simulink model "quadsim2009"  (Simulink 7.7)
settings: Solver=ode45  StartTime=0.0  StopTime=50  RelTol=1e-3
values from neighbouring files (symbols this model uses):
  b = 9.7575e-6    (= 9.7575e-06)    [ForcesTest.m]    (also in QuadDynamics.m = 9.937e-09; QuadDynamicsC.m = 1.7246e-06; Quadparameters.m = 3.13e-05; quadparam.m = 3.13e-05)
  d = 7.5*10^(-7)    (= 7.5e-07)    [Quadparameters.m]    (also in quadparam.m)
  g = 9.81    [ForcesTest.m]    (also in QuadDynamics.m; QuadDynamicsC.m; Quadparameters.m; quadparam.m)
  Ix = 7.5*10^(-3)    (= 0.0075)    [Quadparameters.m]    (also in quadparam.m)
  Iy = 7.5*10^(-3)    (= 0.0075)    [Quadparameters.m]    (also in quadparam.m)
  Iz = 1.3*10^(-2)    (= 0.013)    [Quadparameters.m]    (also in quadparam.m)
  Jr = 6.5*10^(-5)    (= 6.5e-05)    [Quadparameters.m]    (also in quadparam.m = 0.100065)
  kdp = 0.4    [Quadparameters.m]    (also in quadparam.m)
  kdps = 0.4    [Quadparameters.m]    (also in quadparam.m)
  kdt = 0.4    [Quadparameters.m]    (also in quadparam.m)
  kdz = 20    [Quadparameters.m]    (also in quadparam.m = 80)
  kpp = 0.8    [Quadparameters.m]    (also in quadparam.m)
  kpps = 1    [Quadparameters.m]    (also in quadparam.m)
  kpt = 1.2    [Quadparameters.m]    (also in quadparam.m)
  kpz = 100    [Quadparameters.m]    (also in quadparam.m)
  l = 0.3    [ForcesTest.m]    (also in QuadDynamics.m = 0.254; QuadDynamicsC.m = 0.254; Quadparameters.m = 0.23; quadparam.m = 0.5)
  m = 1.282    [ForcesTest.m]    (also in QuadDynamics.m = 1.284; QuadDynamicsC.m = 1.284; Quadparameters.m = 0.65; quadparam.m = 0.65)
libraries: simulink x2
settings Model: Creator=abdelrazzak.merheb  LastModifiedBy=Alexey
settings DebuggingCC: StrictBusMsg=Warning

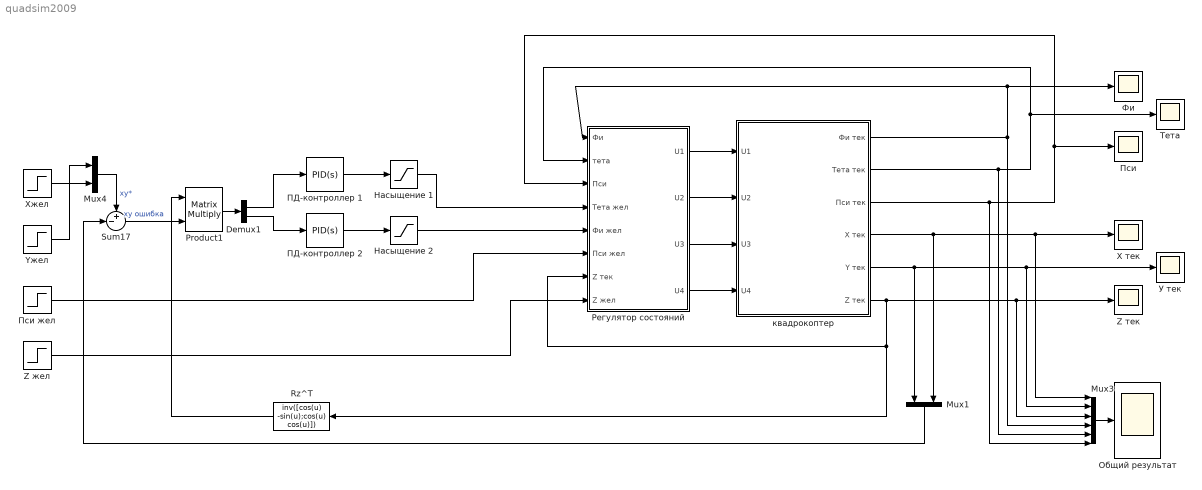
== system quadsim2009 ==
  Demux1 : Demux  Outputs=2
  Mux1 : Mux  Inputs=2
  Mux3 : Mux  Inputs=6
  Mux4 : Mux  Inputs=2
  Product1 : Product  Multiplication=Matrix(*)  RndMeth=Zero
  Rz^T : MATLABFcn  MATLABFcn=inv([cos(u) -sin(u);cos(u) cos(u)])  OutputDimensions=[2 2]  Output1D=off
  Sum17 : Sum  Inputs=+-|
  X тек : Scope
      settings: TimeRange=50  YMin=-0.02  YMax=0.08  SaveName=ScopeData6
  Xжел : Step  Time=10  After=2  SampleTime=0
  Yжел : Step  After=4  SampleTime=0
  Z жел : Step  After=20  SampleTime=0
  Z тек : Scope
      settings: TimeRange=50  YMin=0  YMax=1.4  SaveName=ScopeData4
  Насыщение 1 : Saturate  LinearizeAsGain=off
  Насыщение 2 : Saturate
  Общий результат : Scope
      settings: SaveName=ScopeData3
  ПД-контроллер 1 : simulink/Continuous/PID Controller  SystemSampleTime=-1  Controller=PID  TimeDomain=Continuous-time  SampleTime=1  IntegratorMethod=Forward Euler  FilterMethod=Forward Euler  Form=Parallel  P=1  I=0.1  D=2  N=100  InitialConditionSource=internal  InitialConditionForIntegrator=0  InitialConditionForFilter=0  ExternalReset=none  LimitOutput=off  UpperSaturationLimit=inf  LowerSaturationLimit=-inf  LinearizeAsGain=off  AntiWindupMode=none  Kb=1  TrackingMode=off  Kt=1  PParamMin=[]  PParamMax=[]  IParamMin=[]  IParamMax=[]  DParamMin=[]  DParamMax=[]  NParamMin=[]  NParamMax=[]  KbParamMin=[]  KbParamMax=[]  KtParamMin=[]  KtParamMax=[]  POutMin=[]  POutMax=[]  IOutMin=[]  IOutMax=[]  DOutMin=[]  DOutMax=[]  NOutMin=[]  NOutMax=[]  KbOutMin=[]  KbOutMax=[]  KtOutMin=[]  KtOutMax=[]  IntegratorOutMin=[]  IntegratorOutMax=[]  FilterOutMin=[]  FilterOutMax=[]  SumOutMin=[]  SumOutMax=[]  SumI1OutMin=[]  SumI1OutMax=[]  SumI2OutMin=[]  SumI2OutMax=[]  SumI3OutMin=[]  SumI3OutMax=[]  SumDOutMin=[]  SumDOutMax=[]  SaturationOutMin=[]  SaturationOutMax=[]  IntegratorContinuousStateAttributes=''  IntegratorStateMustResolveToSignalObject=off  IntegratorRTWStateStorageClass=Auto  FilterContinuousStateAttributes=''  FilterStateMustResolveToSignalObject=off  FilterRTWStateStorageClass=Auto
  ПД-контроллер 2 : simulink/Continuous/PID Controller  SystemSampleTime=-1  Controller=PID  TimeDomain=Continuous-time  SampleTime=1  IntegratorMethod=Forward Euler  FilterMethod=Forward Euler  Form=Parallel  P=1  I=0.1  D=2  N=100  InitialConditionSource=internal  InitialConditionForIntegrator=0  InitialConditionForFilter=0  ExternalReset=none  LimitOutput=off  UpperSaturationLimit=inf  LowerSaturationLimit=-inf  LinearizeAsGain=off  AntiWindupMode=none  Kb=1  TrackingMode=off  Kt=1  PParamMin=[]  PParamMax=[]  IParamMin=[]  IParamMax=[]  DParamMin=[]  DParamMax=[]  NParamMin=[]  NParamMax=[]  KbParamMin=[]  KbParamMax=[]  KtParamMin=[]  KtParamMax=[]  POutMin=[]  POutMax=[]  IOutMin=[]  IOutMax=[]  DOutMin=[]  DOutMax=[]  NOutMin=[]  NOutMax=[]  KbOutMin=[]  KbOutMax=[]  KtOutMin=[]  KtOutMax=[]  IntegratorOutMin=[]  IntegratorOutMax=[]  FilterOutMin=[]  FilterOutMax=[]  SumOutMin=[]  SumOutMax=[]  SumI1OutMin=[]  SumI1OutMax=[]  SumI2OutMin=[]  SumI2OutMax=[]  SumI3OutMin=[]  SumI3OutMax=[]  SumDOutMin=[]  SumDOutMax=[]  SaturationOutMin=[]  SaturationOutMax=[]  IntegratorContinuousStateAttributes=''  IntegratorStateMustResolveToSignalObject=off  IntegratorRTWStateStorageClass=Auto  FilterContinuousStateAttributes=''  FilterStateMustResolveToSignalObject=off  FilterRTWStateStorageClass=Auto
  Пси : Scope
      settings: YMin=1.08342  YMax=1.08355
  Пси жел : Step  After=0  SampleTime=0
  Регулятор состояний : Subsystem
  Тета : Scope
      settings: TimeRange=30  YMin=-0.5  YMax=2  SaveName=ScopeData2
  У тек : Scope
      settings: TimeRange=30  YMin=-0.5  YMax=2  SaveName=ScopeData7
  Фи : Scope
      settings: TimeRange=50  YMax=25
  квадрокоптер : Subsystem
  wires:
  Регулятор состояний/1(U1) -> квадрокоптер/1(U1)
  Регулятор состояний/2(U2) -> квадрокоптер/2(U2)
  Регулятор состояний/3(U3) -> квадрокоптер/3(U3)
  Регулятор состояний/4(U4) -> квадрокоптер/4(U4)
  квадрокоптер/6(Z тек) -> Регулятор состояний/7(Z тек), Rz^T/1, Z тек/1, Mux3/3
  квадрокоптер/2(Тета тек) -> Mux3/5, Регулятор состояний/2(тета), Тета/1
  квадрокоптер/3(Пси тек) -> Mux3/6, Регулятор состояний/3(Пси), Пси/1
  Пси жел/1 -> Регулятор состояний/6(Пси жел)
  Z жел/1 -> Регулятор состояний/8(Z жел)
  квадрокоптер/4(X тек) -> Mux1/2, X тек/1, Mux3/1
  квадрокоптер/5(Y тек) -> Mux1/1, У тек/1, Mux3/2
  Mux3/1 -> Общий результат/1
  Yжел/1 -> Mux4/1
  Xжел/1 -> Mux4/2
  Mux4/1 -> Sum17/1  "xy*"
  Rz^T/1 -> Product1/1
  Sum17/1 -> Product1/2  "xy ошибка"
  Product1/1 -> Demux1/1
  Demux1/2 -> ПД-контроллер 2/1
  Demux1/1 -> ПД-контроллер 1/1
  ПД-контроллер 1/1 -> Насыщение 1/1
  ПД-контроллер 2/1 -> Насыщение 2/1
  Mux1/1 -> Sum17/2
  Насыщение 1/1 -> Регулятор состояний/4(Тета жел)
  Насыщение 2/1 -> Регулятор состояний/5(Фи жел)
  квадрокоптер/1(Фи тек) -> Mux3/4, Регулятор состояний/1(Фи), Фи/1

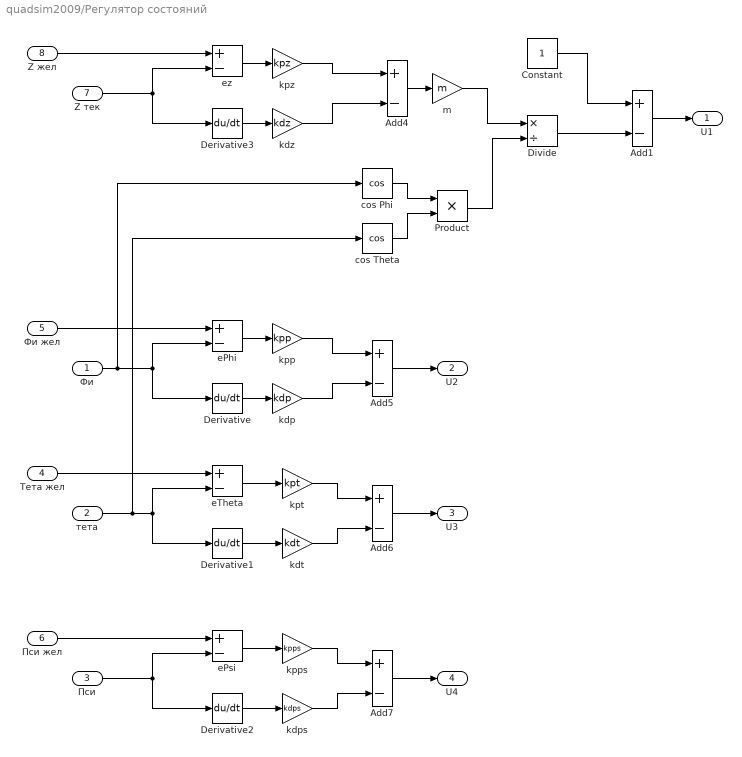
== system quadsim2009/Регулятор состояний ==
  Фи : Inport
  тета : Inport  Port=2
  Пси : Inport  Port=3
  Тета жел : Inport  Port=4
  Фи жел : Inport  Port=5
  Пси жел : Inport  Port=6
  Z тек : Inport  Port=7
  Z жел : Inport  Port=8
  Add{1,4..7} (5 alike) : Sum  Inputs=+-
  Constant : Constant
  Derivative{,1..3} (4 alike) : Derivative
  Divide : Product  Inputs=*/
  Product : Product  RndMeth=Zero
  cos Phi : Trigonometry  Operator=cos
  cos Theta : Trigonometry  Operator=cos
  ePhi : Sum  Inputs=+-
  ePsi : Sum  Inputs=+-
  eTheta : Sum  Inputs=+-
  ez : Sum  Inputs=+-
  kdp : Gain  Gain=kdp
  kdps : Gain  Gain=kdps
  kdt : Gain  Gain=kdt
  kdz : Gain  Gain=kdz
  kpp : Gain  Gain=kpp
  kpps : Gain  Gain=kpps
  kpt : Gain  Gain=kpt
  kpz : Gain  Gain=kpz
  m : Gain  Gain=m
  U1 : Outport
  U2 : Outport  Port=2
  U3 : Outport  Port=3
  U4 : Outport  Port=4
  wires:
  Фи/1 -> Derivative/1, ePhi/2, cos Phi/1
  тета/1 -> Derivative1/1, eTheta/2, cos Theta/1
  Пси/1 -> Derivative2/1, ePsi/2
  Фи жел/1 -> ePhi/1
  Тета жел/1 -> eTheta/1
  Пси жел/1 -> ePsi/1
  ePhi/1 -> kpp/1
  Derivative/1 -> kdp/1
  eTheta/1 -> kpt/1
  Derivative1/1 -> kdt/1
  ePsi/1 -> kpps/1
  Derivative2/1 -> kdps/1
  Z тек/1 -> Derivative3/1, ez/2
  Z жел/1 -> ez/1
  ez/1 -> kpz/1
  Derivative3/1 -> kdz/1
  kpz/1 -> Add4/1
  kdz/1 -> Add4/2
  kpp/1 -> Add5/1
  kdp/1 -> Add5/2
  Add5/1 -> U2/1
  kpt/1 -> Add6/1
  kdt/1 -> Add6/2
  Add6/1 -> U3/1
  kpps/1 -> Add7/1
  kdps/1 -> Add7/2
  Add7/1 -> U4/1
  cos Phi/1 -> Product/1
  cos Theta/1 -> Product/2
  Add4/1 -> m/1
  m/1 -> Divide/1
  Product/1 -> Divide/2
  Constant/1 -> Add1/1
  Divide/1 -> Add1/2
  Add1/1 -> U1/1

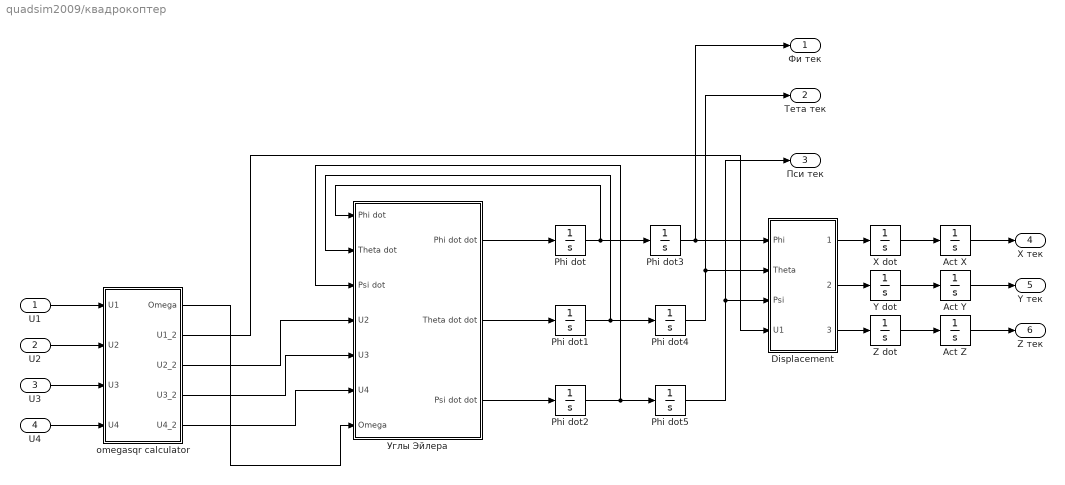
== system quadsim2009/квадрокоптер ==
  U1 : Inport
  U2 : Inport  Port=2
  U3 : Inport  Port=3
  U4 : Inport  Port=4
  Act X : Integrator
  Act Y : Integrator
  Act Z : Integrator
  Displacement : Subsystem
  Phi dot : Integrator
  Phi dot{1..5} (5 alike) : Integrator  ZeroCross=off
  X dot : Integrator
  Y dot : Integrator
  Z dot : Integrator
  omegasqr calculator : Subsystem
  Углы Эйлера : Subsystem
  Фи тек : Outport
  Тета тек : Outport  Port=2
  Пси тек : Outport  Port=3
  X тек : Outport  Port=4
  Y тек : Outport  Port=5
  Z тек : Outport  Port=6
  wires:
  Углы Эйлера/1(Phi dot dot) -> Phi dot/1
  Углы Эйлера/2(Theta dot dot) -> Phi dot1/1
  Углы Эйлера/3(Psi dot dot) -> Phi dot2/1
  Phi dot/1 -> Углы Эйлера/1(Phi dot), Phi dot3/1
  Phi dot1/1 -> Углы Эйлера/2(Theta dot), Phi dot4/1
  Phi dot2/1 -> Углы Эйлера/3(Psi dot), Phi dot5/1
  omegasqr calculator/3(U2_2) -> Углы Эйлера/4(U2)
  omegasqr calculator/4(U3_2) -> Углы Эйлера/5(U3)
  omegasqr calculator/5(U4_2) -> Углы Эйлера/6(U4)
  omegasqr calculator/1(Omega) -> Углы Эйлера/7(Omega)
  Phi dot3/1 -> Displacement/1(Phi), Фи тек/1
  Phi dot4/1 -> Displacement/2(Theta), Тета тек/1
  Phi dot5/1 -> Displacement/3(Psi), Пси тек/1
  omegasqr calculator/2(U1_2) -> Displacement/4(U1)
  Displacement/1(x dotdot) -> X dot/1
  X dot/1 -> Act X/1
  Y dot/1 -> Act Y/1
  Displacement/2(y dotdot) -> Y dot/1
  Z dot/1 -> Act Z/1
  Displacement/3(z dotdot) -> Z dot/1
  Act X/1 -> X тек/1
  Act Y/1 -> Y тек/1
  Act Z/1 -> Z тек/1
  U1/1 -> omegasqr calculator/1(U1)
  U2/1 -> omegasqr calculator/2(U2)
  U3/1 -> omegasqr calculator/3(U3)
  U4/1 -> omegasqr calculator/4(U4)

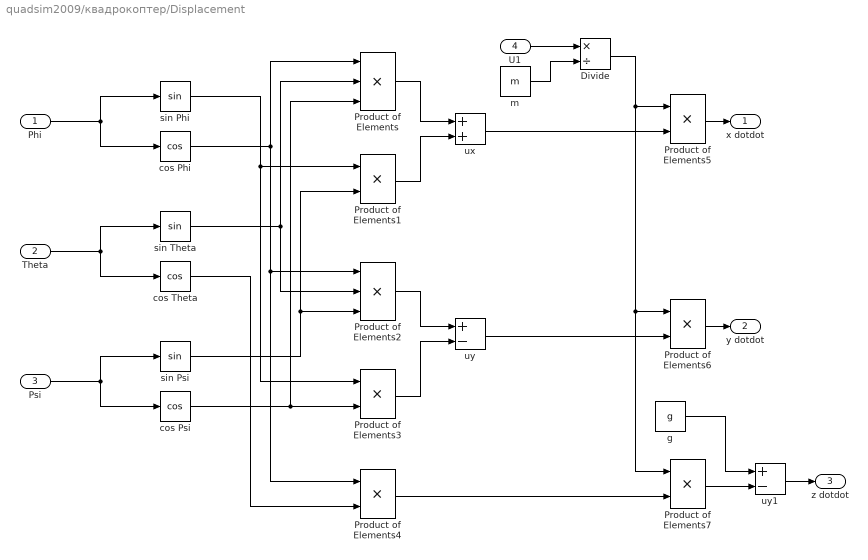
== system quadsim2009/квадрокоптер/Displacement ==
  Phi : Inport
  Theta : Inport  Port=2
  Psi : Inport  Port=3
  U1 : Inport  Port=4
  Divide : Product  Inputs=*/
  Product of Elements : Product  Inputs=3
  Product of Elements{1,3..7} (6 alike) : Product
  Product of Elements2 : Product  Inputs=3
  cos Phi : Trigonometry  Operator=cos
  cos Psi : Trigonometry  Operator=cos
  cos Theta : Trigonometry  Operator=cos
  g : Constant  Value=g
  m : Constant  Value=m
  sin Phi : Trigonometry
  sin Psi : Trigonometry
  sin Theta : Trigonometry
  ux : Sum
  uy : Sum  Inputs=+-
  uy1 : Sum  Inputs=+-
  x dotdot : Outport
  y dotdot : Outport  Port=2
  z dotdot : Outport  Port=3
  wires:
  Phi/1 -> sin Phi/1, cos Phi/1
  Theta/1 -> sin Theta/1, cos Theta/1
  Psi/1 -> sin Psi/1, cos Psi/1
  sin Theta/1 -> Product of Elements/2, Product of Elements2/2
  cos Psi/1 -> Product of Elements/3, Product of Elements3/2
  cos Phi/1 -> Product of Elements/1, Product of Elements2/1, Product of Elements4/1
  sin Phi/1 -> Product of Elements1/1, Product of Elements3/1
  sin Psi/1 -> Product of Elements1/2, Product of Elements2/3
  Product of Elements/1 -> ux/1
  Product of Elements1/1 -> ux/2
  ux/1 -> Product of Elements5/2
  Product of Elements2/1 -> uy/1
  Product of Elements3/1 -> uy/2
  uy/1 -> Product of Elements6/2
  cos Theta/1 -> Product of Elements4/2
  Product of Elements4/1 -> Product of Elements7/2
  U1/1 -> Divide/1
  m/1 -> Divide/2
  Divide/1 -> Product of Elements5/1, Product of Elements6/1, Product of Elements7/1
  Product of Elements5/1 -> x dotdot/1
  Product of Elements6/1 -> y dotdot/1
  uy1/1 -> z dotdot/1
  Product of Elements7/1 -> uy1/2
  g/1 -> uy1/1

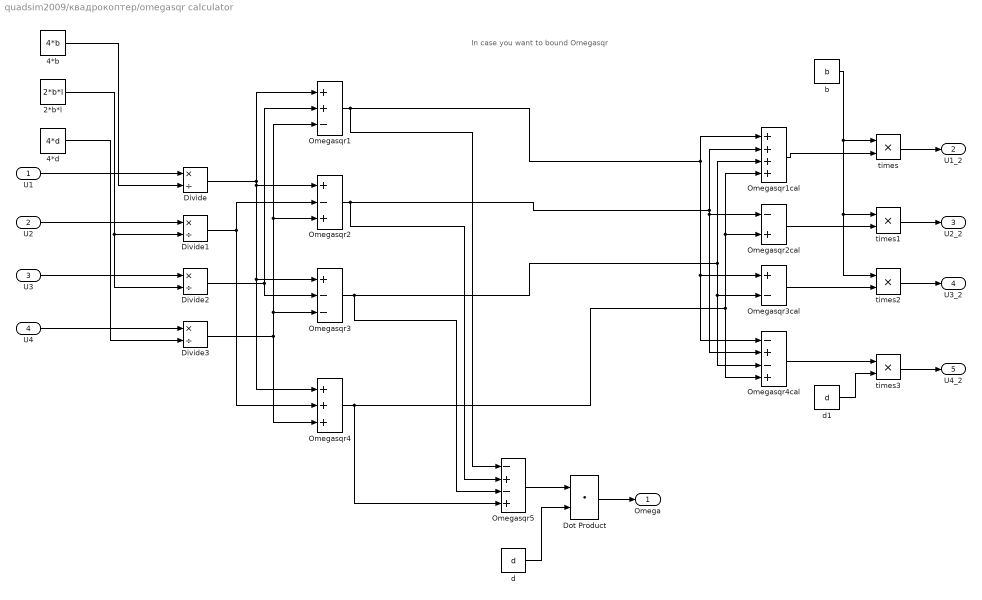
== system quadsim2009/квадрокоптер/omegasqr calculator ==
  note: In case you want to bound Omegasqr
  U1 : Inport
  U2 : Inport  Port=2
  U3 : Inport  Port=3
  U4 : Inport  Port=4
  2*b*l : Constant  Value=2*b*l
  4*b : Constant  Value=4*b
  4*d : Constant  Value=4*d
  Divide{,1..3} (4 alike) : Product  Inputs=*/
  Dot Product : DotProduct  InputSameDT=on  OutDataTypeStr=Inherit: Inherit via internal rule
  Omegasqr1 : Sum  Inputs=++-
  Omegasqr1cal : Sum  Inputs=++++
  Omegasqr2 : Sum  Inputs=+-+
  Omegasqr2cal : Sum  Inputs=-+
  Omegasqr3 : Sum  Inputs=+--
  Omegasqr3cal : Sum  Inputs=+-
  Omegasqr4 : Sum  Inputs=+++
  Omegasqr4cal : Sum  Inputs=-+-+
  Omegasqr5 : Sum  Inputs=-+-+
  b : Constant  Value=b
  d : Constant  Value=d
  d1 : Constant  Value=d
  times{,1..3} (4 alike) : Product  Inputs=**
  Omega : Outport
  U1_2 : Outport  Port=2
  U2_2 : Outport  Port=3
  U3_2 : Outport  Port=4
  U4_2 : Outport  Port=5
  wires:
  U1/1 -> Divide/1
  4*b/1 -> Divide/2
  U2/1 -> Divide1/1
  2*b*l/1 -> Divide1/2, Divide2/2
  U3/1 -> Divide2/1
  U4/1 -> Divide3/1
  4*d/1 -> Divide3/2
  Divide/1 -> Omegasqr1/1, Omegasqr2/1, Omegasqr3/1, Omegasqr4/1
  Divide2/1 -> Omegasqr1/2, Omegasqr3/2
  Divide3/1 -> Omegasqr1/3, Omegasqr2/3, Omegasqr3/3, Omegasqr4/3
  Divide1/1 -> Omegasqr2/2, Omegasqr4/2
  Omegasqr1/1 -> Omegasqr5/1, Omegasqr1cal/1, Omegasqr3cal/1, Omegasqr4cal/1
  Omegasqr2/1 -> Omegasqr5/2, Omegasqr1cal/2, Omegasqr2cal/1, Omegasqr4cal/2
  Omegasqr3/1 -> Omegasqr5/3, Omegasqr1cal/3, Omegasqr3cal/2, Omegasqr4cal/3
  Omegasqr4/1 -> Omegasqr5/4, Omegasqr1cal/4, Omegasqr2cal/2, Omegasqr4cal/4
  Omegasqr5/1 -> Dot Product/1
  Dot Product/1 -> Omega/1
  d/1 -> Dot Product/2
  b/1 -> times/1, times1/1, times2/1
  Omegasqr1cal/1 -> times/2
  Omegasqr2cal/1 -> times1/2
  Omegasqr3cal/1 -> times2/2
  Omegasqr4cal/1 -> times3/1
  d1/1 -> times3/2
  times/1 -> U1_2/1
  times1/1 -> U2_2/1
  times3/1 -> U4_2/1
  times2/1 -> U3_2/1

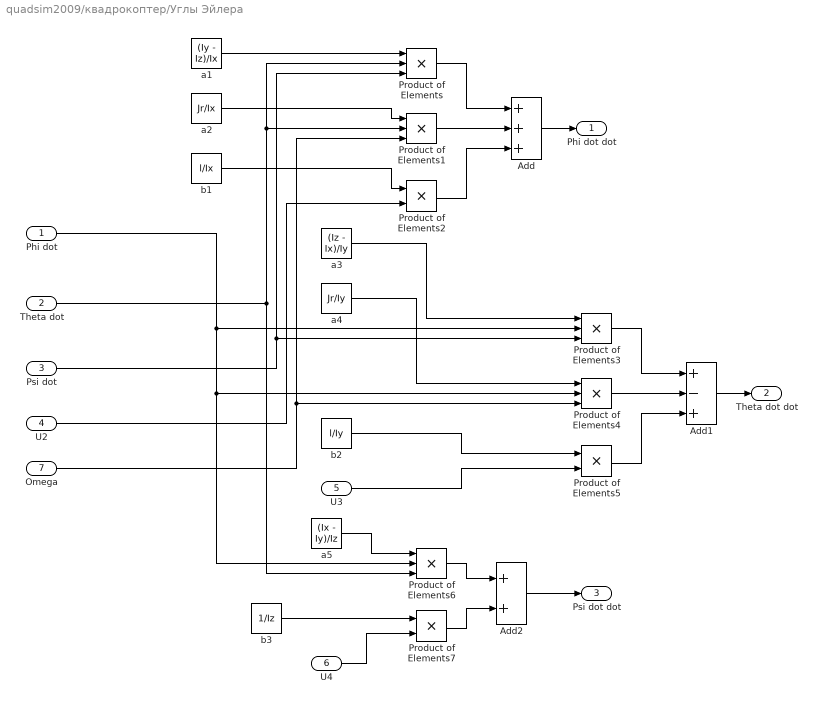
== system quadsim2009/квадрокоптер/Углы Эйлера ==
  Phi dot : Inport
  Theta dot : Inport  Port=2
  Psi dot : Inport  Port=3
  U2 : Inport  Port=4
  U3 : Inport  Port=5
  U4 : Inport  Port=6
  Omega : Inport  Port=7
  Add : Sum  Inputs=+++
  Add1 : Sum  Inputs=+-+
  Add2 : Sum
  Product of Elements{,1,3..4,6} (5 alike) : Product  Inputs=3
  Product of Elements2 : Product
  Product of Elements5 : Product
  Product of Elements7 : Product
  a1 : Constant  Value=(Iy - Iz)/Ix
  a2 : Constant  Value=Jr/Ix
  a3 : Constant  Value=(Iz - Ix)/Iy
  a4 : Constant  Value=Jr/Iy
  a5 : Constant  Value=(Ix - Iy)/Iz
  b1 : Constant  Value=l/Ix
  b2 : Constant  Value=l/Iy
  b3 : Constant  Value=1/Iz
  Phi dot dot : Outport
  Theta dot dot : Outport  Port=2
  Psi dot dot : Outport  Port=3
  wires:
  Product of Elements/1 -> Add/1
  Product of Elements1/1 -> Add/2
  Product of Elements2/1 -> Add/3
  Add/1 -> Phi dot dot/1
  a1/1 -> Product of Elements/1
  Theta dot/1 -> Product of Elements/2, Product of Elements1/2, Product of Elements6/3
  Psi dot/1 -> Product of Elements/3, Product of Elements3/3
  a2/1 -> Product of Elements1/1
  b1/1 -> Product of Elements2/1
  U2/1 -> Product of Elements2/2
  Omega/1 -> Product of Elements1/3, Product of Elements4/3
  Product of Elements3/1 -> Add1/1
  Product of Elements4/1 -> Add1/2
  Product of Elements5/1 -> Add1/3
  Add1/1 -> Theta dot dot/1
  a3/1 -> Product of Elements3/1
  a4/1 -> Product of Elements4/1
  b2/1 -> Product of Elements5/1
  U3/1 -> Product of Elements5/2
  Phi dot/1 -> Product of Elements3/2, Product of Elements4/2, Product of Elements6/2
  Product of Elements6/1 -> Add2/1
  Product of Elements7/1 -> Add2/2
  Add2/1 -> Psi dot dot/1
  U4/1 -> Product of Elements7/2
  b3/1 -> Product of Elements7/1
  a5/1 -> Product of Elements6/1
